simulink model "D2C_simulation_boucle_position_0"  (R2016b)
settings: Solver=ode45  StartTime=0.0  StopTime=20  FixedStep=0.003  RelTol=1e-3  EnableMultiTasking=on
libraries: slctrlblks x2
settings Model: Creator=Propriétaire  LastModifiedBy=emiliendurif
settings DataIOCC: LimitDataPoints=on  SaveFormat=Array  SignalLoggingSaveFormat=ModelDataLogs
settings OptimizationCC: ExpressionDepthLimit=2147483647  LifeSpan=inf
settings DebuggingCC: UnderspecifiedInitializationDetection=Classic  MergeDetectMultiDrivingBlocksExec=none  SolverPrmCheckMsg=warning  FcnCallInpInsideContextMsg=warning  StateNameClashWarn=warning  SFUnexpectedBacktrackingDiag=warning  SFNoUnconditionalDefaultTransitionDiag=warning  SFExecutionAtInitializationDiag=none
settings HardwareCC: ProdBitPerPointer=32  ProdBitPerSizeT=32  ProdBitPerPtrDiffT=32  ProdLargestAtomicFloat=None  ProdIntDivRoundTo=Undefined  ProdEndianess=Unspecified  ProdWordSize=32  ProdHWDeviceType=32-bit Generic
settings ModelReferenceCC: PropagateSignalLabelsOutOfModel=off
settings GRTTargetCC: TargetLangStandard=C89/C90 (ANSI)  GeneratePreprocessorConditionals=Disable all  CombineOutputUpdateFcns=off  GRTInterface=on
settings ConfigComp: CovMetricSettings=dw  CovHtmlReporting=on  CovSaveCumulativeToWorkspaceVar=on  CovSaveSingleToWorkspaceVar=on  CovExternalEMLEnable=off

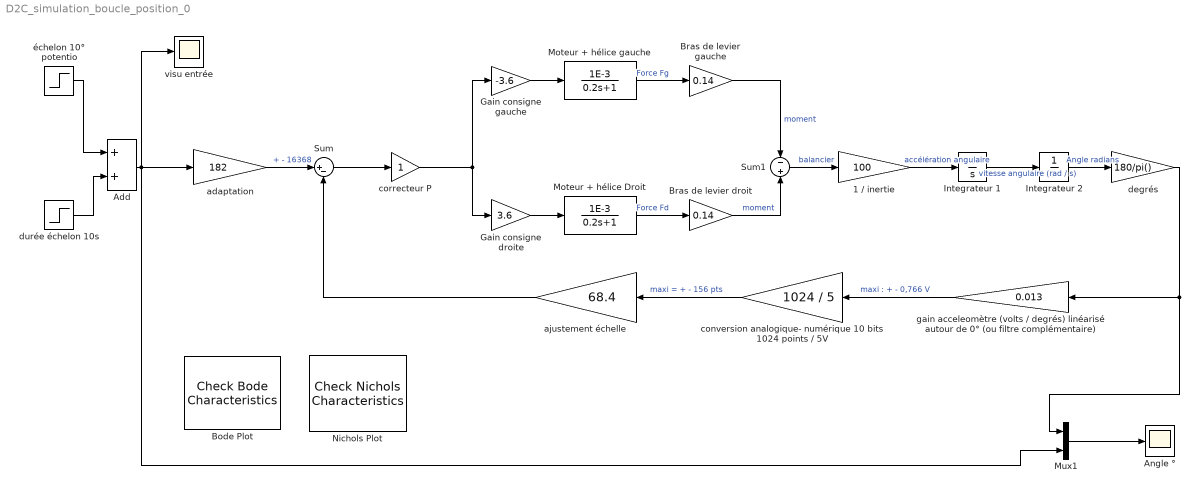
== system D2C_simulation_boucle_position_0 ==
  1 / inertie : Gain  Gain=100
  Add : Sum
  Angle ° : Scope
  Bode Plot : slctrlblks/Model Verification/Check Bode  Characteristics  InstantiateOnLoad=on  SaveOperatingPoints=off  LinearizationIOs={'/Sum', 1, 'in', 'on', '';'/ajustement échelle', 1, 'out', 'on', ''}  LinearizeAt=SnapshotTimes  SnapshotTimes=[0]  TriggerType=rising  SampleTime=auto  RateConversionMethod=zoh  PreWarpFreq=10  UseExactDelayModel=off  UseFullBlockNameLabels=off  UseBusSignalLabels=off  enabled=on  stopWhenAssertionFail=off  export=off  ViewDlgPos=[1492 30 510 390]  OpenViewOnLoad=on  LaunchViewOnOpen=on  FrequencyUnits=rad/s  MagnitudeUnits=dB  PhaseUnits=deg  TimeUnits=seconds  EnableUpperBound=off  UpperBoundFrequencies=[]  UpperBoundMagnitudes=[]  EnableLowerBound=off  LowerBoundFrequencies=[]  LowerBoundMagnitudes=[]
  Bras de levier droit : Gain  Gain=0.14
  Bras de levier gauche : Gain  Gain=0.14
  Gain consigne droite : Gain  Gain=3.6
  Gain consigne gauche : Gain  Gain=-3.6
  Integrateur 1 : Integrator
  Integrateur 2 : Integrator
  Moteur + hélice Droit : TransferFcn  Numerator=[1E-3]  Denominator=[0.2 1]
  Moteur + hélice gauche : TransferFcn  Numerator=[1E-3]  Denominator=[0.2 1]
  Mux1 : Mux  Inputs=2
  Nichols Plot : slctrlblks/Model Verification/Check Nichols Characteristics  InstantiateOnLoad=on  SaveOperatingPoints=off  LinearizationIOs={'/Sum', 1, 'in', 'on', '';'/ajustement échelle', 1, 'out', 'on', ''}  LinearizeAt=SnapshotTimes  SnapshotTimes=[0]  TriggerType=rising  SampleTime=auto  RateConversionMethod=zoh  PreWarpFreq=10  UseExactDelayModel=off  UseFullBlockNameLabels=off  UseBusSignalLabels=off  enabled=on  stopWhenAssertionFail=off  export=off  ViewDlgPos=[1345 245 510 390]  LaunchViewOnOpen=on  OpenViewOnLoad=on  FrequencyUnits=rad/s  MagnitudeUnits=dB  PhaseUnits=deg  TimeUnits=seconds  EnableMargins=off  GainMargin=[]  PhaseMargin=[]  EnableGainPhaseBound=off  GainPhaseBoundType={'upper'}  OLPhases=[]  OLGains=[]  EnableCLPeakGain=off  CLPeakGain=[]  FeedbackSign=-1
      settings: SaveToWorkspace=off  SaveName=sys
  Sum : Sum  Inputs=|+-
  Sum1 : Sum  Inputs=-|+
  adaptation : Gain  Gain=182
  ajustement échelle : Gain  Gain=68.4
  conversion analogique- numérique 10 bits 1024 points / 5V : Gain  Gain=1024 / 5
  correcteur P : Gain
  degrés : Gain  Gain=180/pi()
  durée échelon 10s : Step  Time=10  After=-10  SampleTime=0
  gain acceleomètre (volts / degrés) linéarisé autour de 0° (ou filtre complémentaire) : Gain  Gain=0.013
  visu entrée : Scope
  échelon 10° potentio : Step  Time=0  After=10  SampleTime=0
  wires:
  Moteur + hélice gauche/1 -> Bras de levier gauche/1  "Force Fg"
  Bras de levier gauche/1 -> Sum1/1  "moment"
  Moteur + hélice Droit/1 -> Bras de levier droit/1  "Force Fd"
  Bras de levier droit/1 -> Sum1/2  "moment"
  Gain consigne gauche/1 -> Moteur + hélice gauche/1
  Gain consigne droite/1 -> Moteur + hélice Droit/1
  Sum1/1 -> 1 / inertie/1  "balancier"
  gain acceleomètre (volts / degrés) linéarisé autour de 0° (ou filtre complémentaire)/1 -> conversion analogique- numérique 10 bits 1024 points / 5V/1  "maxi : + - 0,766 V"
  Integrateur 2/1 -> degrés/1  "Angle radians"
  1 / inertie/1 -> Integrateur 1/1  "accélération angulaire"
  Integrateur 1/1 -> Integrateur 2/1  "vitesse angulaire (rad / s)"
  adaptation/1 -> Sum/1  "+ - 16368"
  degrés/1 -> Mux1/1, gain acceleomètre (volts / degrés) linéarisé autour de 0° (ou filtre complémentaire)/1
  Add/1 -> Mux1/2, adaptation/1, visu entrée/1
  échelon 10° potentio/1 -> Add/1
  durée échelon 10s/1 -> Add/2
  conversion analogique- numérique 10 bits 1024 points / 5V/1 -> ajustement échelle/1  "maxi = + - 156 pts"
  Mux1/1 -> Angle °/1
  correcteur P/1 -> Gain consigne droite/1, Gain consigne gauche/1
  ajustement échelle/1 -> Sum/2
  Sum/1 -> correcteur P/1
